simulink library "tire"  (R2025b)
settings: Solver=VariableStepAuto  StartTime=0.0  StopTime=10.0  RelTol=1e-3
settings Model: Creator=jessi  LastModifiedBy=jessi

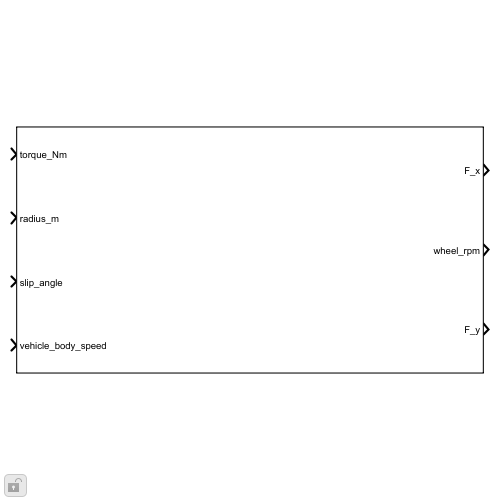
[thumbnail: Simulink's stored preview of the top-level diagram]
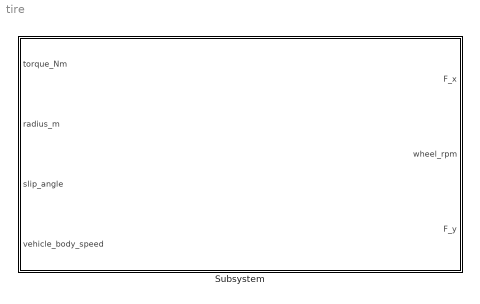
== system tire ==
  Subsystem : Subsystem

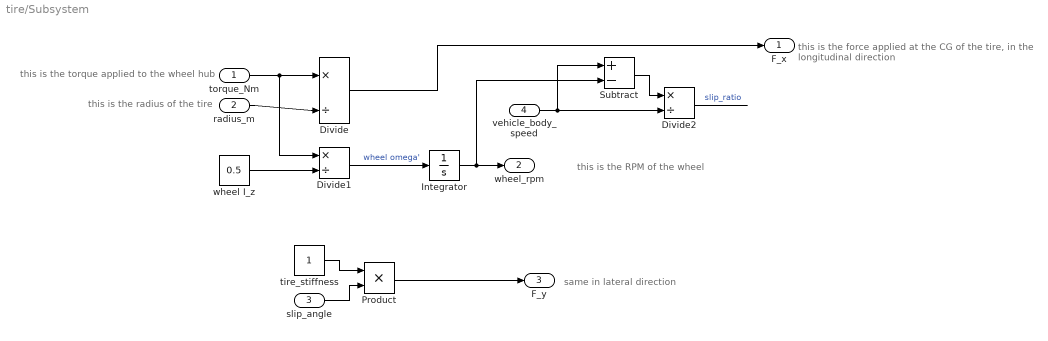
== system tire/Subsystem ==
  note: same in lateral direction
  note: this is the RPM of the wheel
  note: this is the force applied at the CG of the tire, in the longitudinal direction
  note: this is the radius of the tire
  note: this is the torque applied to the wheel hub
  torque_Nm : Inport  Unit=N*m  PortDimensions=4
  radius_m : Inport  Port=2  Unit=m
  slip_angle : Inport  Port=3
  vehicle_body_speed : Inport  Port=4
  Divide : Product  Inputs=*/
  Divide1 : Product  Inputs=*/
  Divide2 : Product  Inputs=*/
  Integrator : Integrator
  Product : Product
  Subtract : Sum  Inputs=+-
  tire_stiffness : Constant
  wheel I_z : Constant  Value=0.5
  F_x : Outport  Unit=N  PortDimensions=4
  wheel_rpm : Outport  Port=2  Unit=rpm  PortDimensions=4
  F_y : Outport  Port=3  Unit=N  PortDimensions=4
  wires:
  Divide/1 -> F_x/1
  radius_m/1 -> Divide/2
  torque_Nm/1 -> Divide1/1, Divide/1
  wheel I_z/1 -> Divide1/2
  Divide1/1 -> Integrator/1  "wheel omega'"
  Integrator/1 -> wheel_rpm/1, Subtract/2
  slip_angle/1 -> Product/2
  tire_stiffness/1 -> Product/1
  Product/1 -> F_y/1
  vehicle_body_speed/1 -> Subtract/1, Divide2/2
  Subtract/1 -> Divide2/1
  Divide2/1 -> ?  "slip_ratio"
